simulink model "simulation"  (R2023b)
settings: Solver=VariableStepAuto  StartTime=0.0  StopTime=3.3  RelTol=1e-3
InitFcn:
  | k=0.0032;
  | q=1.6*10^-19;
  | K=1.38*10^-23;
  | n=1.3;
  | Eg0=1.38e-23;
  | Rs=0.221;
  | Rsh=415.405;
  | Tn=298;
  | Voc=32.9;
  | Isc=8.21;
  | Ns=54;
libraries: simulink x1
settings Model: Creator=aditi  LastModifiedBy=aditi
settings DebuggingCC: AlgebraicLoopMsg=none

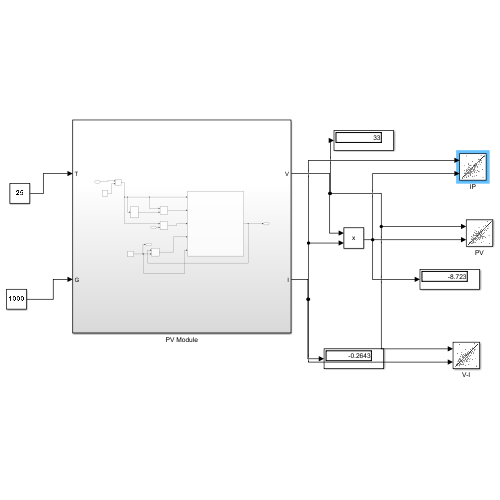
[thumbnail: Simulink's stored preview of the top-level diagram]
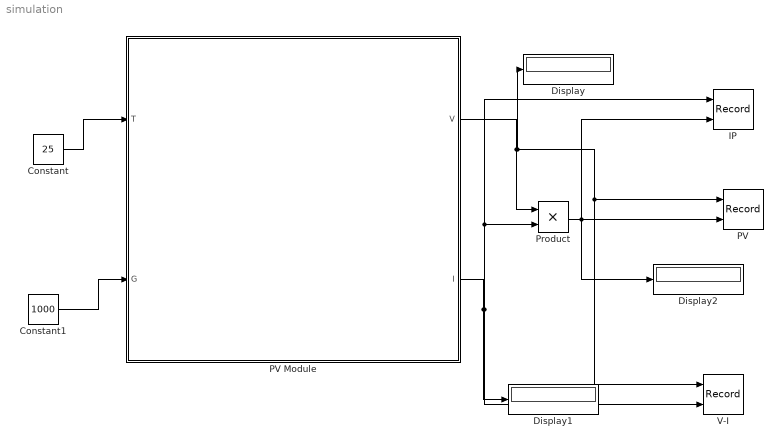
== system simulation ==
  Constant : Constant  Value=25
  Constant1 : Constant  Value=1000
  Display : Display
  Display1 : Display
  Display2 : Display
  IP : Record  FileSettingsInternal="{\"entries\":[{\"content\":{\"excelSettings\":{\"content\":{},\"type\":\"Streamout.ExcelSettings\"}},\"type\":\"Streamout.FileSettingStorage\",\"uuid\":\"\"}],\"packageUris\":[\"http:\\/\\/schema.mathworks.com\\/mf0\\/streamout_blocks\\/R2020a\"],\"version\":\"1.0\"}"  Layout=[1 1]  SignalsInternal="{\"entries\":[{\"content\":{\"signals\":[{\"content\":{\"blockPath\":[],\"dimensions\":[1],\"domain\":\"\",\"lineColor\":\"#77ac30\",\"plots\":[1],\"port\":1,\"sid\":[\"\"],\"signalID\":35,\"signalName\":\"PV Module:2\"},\"type\":\"RecordBlkView.Signal\",\"uuid\":\"\"},{\"content\":{\"blockPath\":[],\"dimensions\":[1],\"domain\":\"\",\"lineColor\":\"#4dbeee\",\"plots\":[1],\"port\":2,\"sid\":[\"\"],\"signalID\":39,\"signalName\":\"Product\"},\"type\":\"RecordBlkView.Signal\",\"uuid\":\"\"}]},\"type\":\"RecordBlkView.InputSignals\",\"uuid\":\"\"}],\"packageUris\":[\"http:\\/\\/schema.mathworks.com\\/mf0\\/streamout_blocks\\/R2020a\"],\"version\":\"1.0\"}"  VisualizationBindings="{\"xyplotplugin\":{\"info\":[{\"series\":[{\"bindingParametersList\":[{\"parameter\":\"X-Axis\",\"signalID\":35,\"signalName\":\"PV Module:2\"},{\"parameter\":\"Y-Axis\",\"signalID\":39,\"signalName\":\"Product\"}],\"seriesID\":19355}],\"subplotID\":1}]}}"  CompatibilityTag=XY  st=-1
  PV : Record  FileSettingsInternal="{\"entries\":[{\"content\":{\"excelSettings\":{\"content\":{},\"type\":\"Streamout.ExcelSettings\"}},\"type\":\"Streamout.FileSettingStorage\",\"uuid\":\"\"}],\"packageUris\":[\"http:\\/\\/schema.mathworks.com\\/mf0\\/streamout_blocks\\/R2020a\"],\"version\":\"1.0\"}"  Layout=[1 1]  SignalsInternal="{\"entries\":[{\"content\":{\"signals\":[{\"content\":{\"blockPath\":[],\"dimensions\":[1],\"domain\":\"\",\"lineColor\":\"#77ac30\",\"plots\":[1],\"port\":1,\"sid\":[\"\"],\"signalID\":43,\"signalName\":\"PV Module:1\"},\"type\":\"RecordBlkView.Signal\",\"uuid\":\"\"},{\"content\":{\"blockPath\":[],\"dimensions\":[1],\"domain\":\"\",\"lineColor\":\"#4dbeee\",\"plots\":[1],\"port\":2,\"sid\":[\"\"],\"signalID\":47,\"signalName\":\"Product\"},\"type\":\"RecordBlkView.Signal\",\"uuid\":\"\"}]},\"type\":\"RecordBlkView.InputSignals\",\"uuid\":\"\"}],\"packageUris\":[\"http:\\/\\/schema.mathworks.com\\/mf0\\/streamout_blocks\\/R2020a\"],\"version\":\"1.0\"}"  VisualizationBindings="{\"xyplotplugin\":{\"info\":[{\"series\":[{\"bindingParametersList\":[{\"parameter\":\"X-Axis\",\"signalID\":43,\"signalName\":\"PV Module:1\"},{\"parameter\":\"Y-Axis\",\"signalID\":47,\"signalName\":\"Product\"}],\"seriesID\":25385}],\"subplotID\":1}]}}"  CompatibilityTag=XY  st=-1
  PV Module : Subsystem
  Product : Product
  V-I : Record  FileSettingsInternal="{\"entries\":[{\"content\":{\"excelSettings\":{\"content\":{},\"type\":\"Streamout.ExcelSettings\"}},\"type\":\"Streamout.FileSettingStorage\",\"uuid\":\"\"}],\"packageUris\":[\"http:\\/\\/schema.mathworks.com\\/mf0\\/streamout_blocks\\/R2020a\"],\"version\":\"1.0\"}"  Layout=[1 1]  SignalsInternal="{\"entries\":[{\"content\":{\"signals\":[{\"content\":{\"blockPath\":[],\"dimensions\":[1],\"domain\":\"\",\"lineColor\":\"#a2142f\",\"plots\":[1],\"port\":1,\"sid\":[\"\"],\"signalID\":51,\"signalName\":\"PV Module:1\"},\"type\":\"RecordBlkView.Signal\",\"uuid\":\"\"},{\"content\":{\"blockPath\":[],\"dimensions\":[1],\"domain\":\"\",\"lineColor\":\"#139fff\",\"plots\":[1],\"port\":2,\"sid\":[\"\"],\"signalID\":55,\"signalName\":\"PV Module:2\"},\"type\":\"RecordBlkView.Signal\",\"uuid\":\"\"}]},\"type\":\"RecordBlkView.InputSignals\",\"uuid\":\"\"}],\"packageUris\":[\"http:\\/\\/schema.mathworks.com\\/mf0\\/streamout_blocks\\/R2020a\"],\"version\":\"1.0\"}"  VisualizationBindings="{\"xyplotplugin\":{\"info\":[{\"series\":[{\"bindingParametersList\":[{\"parameter\":\"Y-Axis\",\"signalID\":55,\"signalName\":\"PV Module:2\"},{\"parameter\":\"X-Axis\",\"signalID\":51,\"signalName\":\"PV Module:1\"}],\"seriesID\":21075}],\"subplotID\":1}]}}"  CompatibilityTag=XY  st=-1
  wires:
  Constant1/1 -> PV Module/2(G)
  Constant/1 -> PV Module/1(T)
  PV Module/1(V) -> Product/1, Display/1, V-I/1, PV/1
  PV Module/2(I) -> Display1/1, IP/1, Product/2, V-I/2
  Product/1 -> IP/2, PV/2, Display2/1

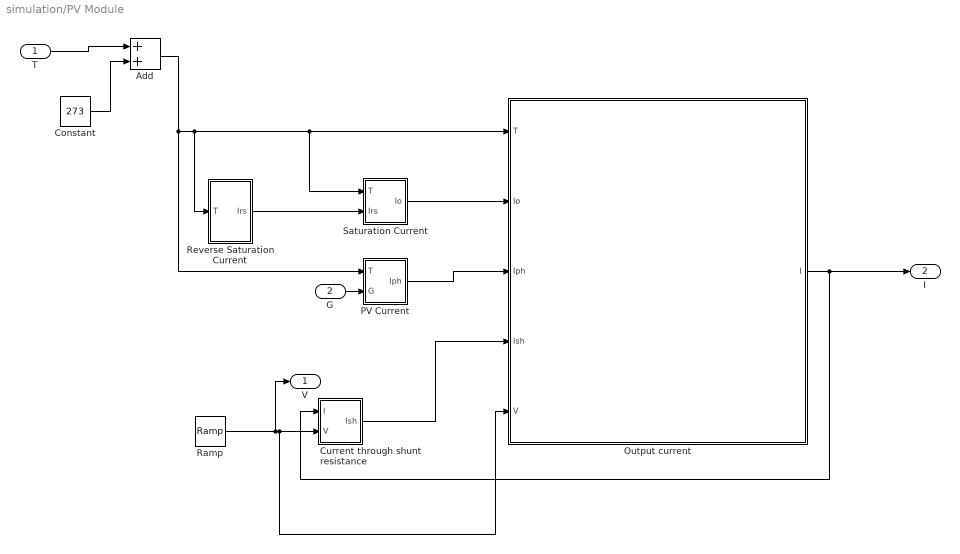
== system simulation/PV Module ==
  T : Inport
  G : Inport  Port=2
  Add : Sum
  Constant : Constant  Value=273
  Current through shunt resistance : Subsystem
  Output current : Subsystem
  PV Current : Subsystem
  Ramp : simulink/Sources/Ramp  slope=10  start=0  InitialOutput=0
  Reverse Saturation Current : Subsystem
  Saturation Current : Subsystem
  V : Outport
  I : Outport  Port=2
  wires:
  Reverse Saturation Current/1(Irs) -> Saturation Current/2(Irs)
  Constant/1 -> Add/2
  Ramp/1 -> V/1, Current through shunt resistance/2(V), Output current/5(V)
  Add/1 -> PV Current/1(T), Reverse Saturation Current/1(T), Saturation Current/1(T), Output current/1(T)
  Current through shunt resistance/1(Ish) -> Output current/4(Ish)
  Saturation Current/1(Io) -> Output current/2(Io)
  PV Current/1(Iph) -> Output current/3(Iph)
  Output current/1(I) -> I/1, Current through shunt resistance/1(I)
  T/1 -> Add/1
  G/1 -> PV Current/2(G)

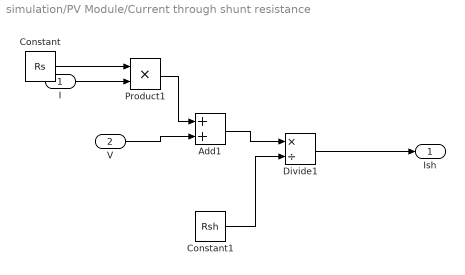
== system simulation/PV Module/Current through shunt resistance ==
  I : Inport
  V : Inport  Port=2
  Add1 : Sum
  Constant : Constant  Value=Rs
  Constant1 : Constant  Value=Rsh
  Divide1 : Product  Inputs=*/
  Product1 : Product
  Ish : Outport
  wires:
  Product1/1 -> Add1/1
  Constant/1 -> Product1/1
  Add1/1 -> Divide1/1
  Constant1/1 -> Divide1/2
  V/1 -> Add1/2
  I/1 -> Product1/2
  Divide1/1 -> Ish/1

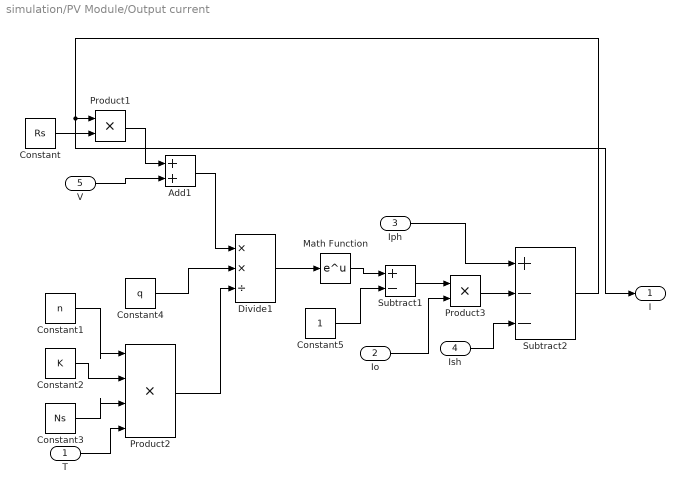
== system simulation/PV Module/Output current ==
  T : Inport
  Io : Inport  Port=2
  Iph : Inport  Port=3
  Ish : Inport  Port=4
  V : Inport  Port=5
  Add1 : Sum
  Constant : Constant  Value=Rs
  Constant1 : Constant  Value=n
  Constant2 : Constant  Value=K
  Constant3 : Constant  Value=Ns
  Constant4 : Constant  Value=q
  Constant5 : Constant
  Divide1 : Product  Inputs=**/
  Math Function : Math
  Product1 : Product
  Product2 : Product  Inputs=4
  Product3 : Product
  Subtract1 : Sum  Inputs=+-
  Subtract2 : Sum  Inputs=+--
  I : Outport
  wires:
  Product2/1 -> Divide1/3
  Constant5/1 -> Subtract1/2
  Constant3/1 -> Product2/3
  Math Function/1 -> Subtract1/1
  Constant2/1 -> Product2/2
  Ish/1 -> Subtract2/3
  Product1/1 -> Add1/1
  Constant4/1 -> Divide1/2
  Add1/1 -> Divide1/1
  Constant/1 -> Product1/2
  Product3/1 -> Subtract2/2
  Subtract2/1 -> I/1, Product1/1
  Divide1/1 -> Math Function/1
  Subtract1/1 -> Product3/1
  Constant1/1 -> Product2/1
  T/1 -> Product2/4
  Iph/1 -> Subtract2/1
  Io/1 -> Product3/2
  V/1 -> Add1/2

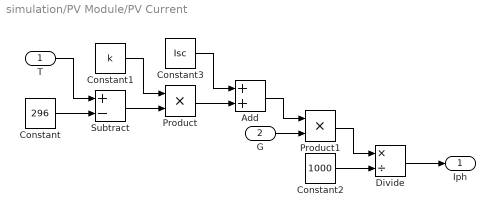
== system simulation/PV Module/PV Current ==
  T : Inport
  G : Inport  Port=2
  Add : Sum
  Constant : Constant  Value=296
  Constant1 : Constant  Value=k
  Constant2 : Constant  Value=1000
  Constant3 : Constant  Value=Isc
  Divide : Product  Inputs=*/
  Product : Product
  Product1 : Product
  Subtract : Sum  Inputs=+-
  Iph : Outport
  wires:
  Add/1 -> Product1/1
  T/1 -> Subtract/1
  Constant/1 -> Subtract/2
  G/1 -> Product1/2
  Constant3/1 -> Add/1
  Constant1/1 -> Product/1
  Subtract/1 -> Product/2
  Product/1 -> Add/2
  Product1/1 -> Divide/1
  Constant2/1 -> Divide/2
  Divide/1 -> Iph/1

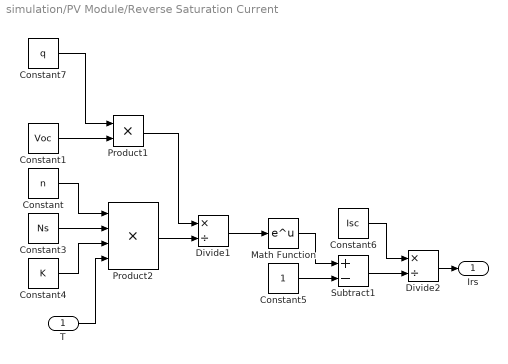
== system simulation/PV Module/Reverse Saturation Current ==
  T : Inport
  Constant : Constant  Value=n
  Constant1 : Constant  Value=Voc
  Constant3 : Constant  Value=Ns
  Constant4 : Constant  Value=K
  Constant5 : Constant
  Constant6 : Constant  Value=Isc
  Constant7 : Constant  Value=q
  Divide1 : Product  Inputs=*/
  Divide2 : Product  Inputs=*/
  Math Function : Math
  Product1 : Product
  Product2 : Product  Inputs=4
  Subtract1 : Sum  Inputs=+-
  Irs : Outport
  wires:
  Constant6/1 -> Divide2/1
  Math Function/1 -> Subtract1/1
  Constant/1 -> Product2/1
  Product2/1 -> Divide1/2
  Constant7/1 -> Product1/1
  Constant3/1 -> Product2/2
  Product1/1 -> Divide1/1
  Constant4/1 -> Product2/3
  Constant1/1 -> Product1/2
  Divide1/1 -> Math Function/1
  Constant5/1 -> Subtract1/2
  Subtract1/1 -> Divide2/2
  Divide2/1 -> Irs/1
  T/1 -> Product2/4

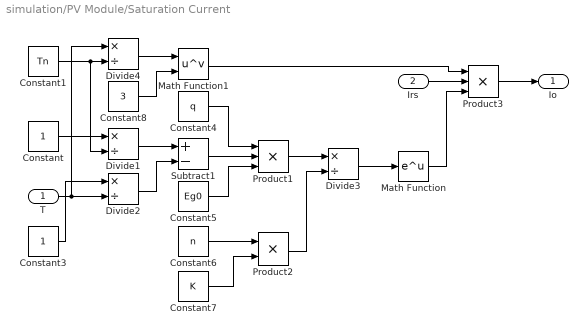
== system simulation/PV Module/Saturation Current ==
  T : Inport
  Irs : Inport  Port=2
  Constant : Constant
  Constant1 : Constant  Value=Tn
  Constant3 : Constant
  Constant4 : Constant  Value=q
  Constant5 : Constant  Value=Eg0
  Constant6 : Constant  Value=n
  Constant7 : Constant  Value=K
  Constant8 : Constant  Value=3
  Divide{1..4} (4 alike) : Product  Inputs=*/
  Math Function : Math
  Math Function1 : Math  Operator=pow
  Product1 : Product  Inputs=3
  Product2 : Product
  Product3 : Product  Inputs=3
  Subtract1 : Sum  Inputs=+-
  Io : Outport
  wires:
  Constant1/1 -> Divide1/2, Divide4/2
  Constant/1 -> Divide1/1
  T/1 -> Divide2/2, Divide4/1
  Constant8/1 -> Math Function1/2
  Divide4/1 -> Math Function1/1
  Constant3/1 -> Divide2/1
  Divide1/1 -> Subtract1/1
  Divide2/1 -> Subtract1/2
  Math Function1/1 -> Product3/1
  Constant4/1 -> Product1/1
  Subtract1/1 -> Product1/2
  Constant5/1 -> Product1/3
  Constant6/1 -> Product2/1
  Constant7/1 -> Product2/2
  Product1/1 -> Divide3/1
  Product2/1 -> Divide3/2
  Divide3/1 -> Math Function/1
  Irs/1 -> Product3/2
  Math Function/1 -> Product3/3
  Product3/1 -> Io/1
